simulink model "MPSK_AWGN"  (R2013a)
settings: Solver=ode45  StartTime=0.0  StopTime=10.0  RelTol=1e-3
values from neighbouring files (symbols this model uses):
  EbNodB = EbNoVec(n)    [PSK_AWGN.m]
  M = 8    [PSK_AWGN.m]    (also in SimulatePSK.m = 2.^k; Untitled2.m)
  Tsym = 0.1    [PSK_AWGN.m]
libraries: commsink2 x2, commutil2 x2, commdigbbndpm3 x2, commchan3 x1, commrandsrc2 x1
settings Model: Creator=Administrator  LastModifiedBy=Administrator

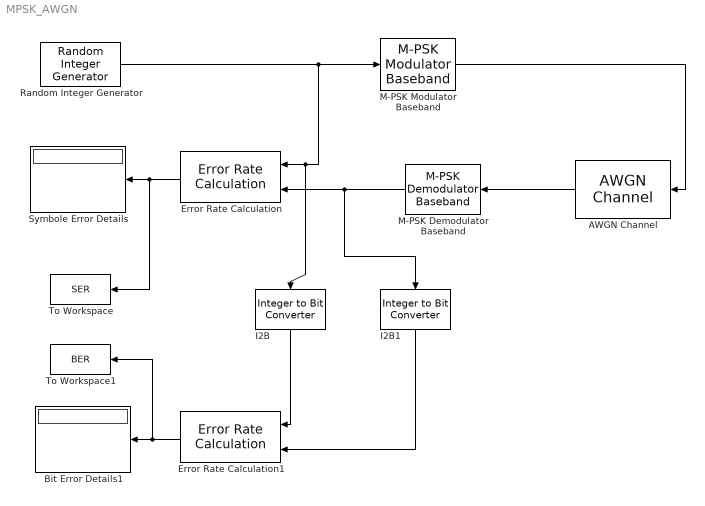
== system MPSK_AWGN ==
  AWGN Channel : commchan3/AWGN Channel  InputProcessing=Columns as channels (frame based)  seed=123456  noiseMode="Signal to noise ratio  (Eb/No)"  EbNodB=EbNodB+10*log10(log2(M))  EsNodB=10  SNRdB=10  bitsPerSym=1  Ps=1  Tsym=Tsym  variance=1
  Bit Error Details1 : Display
      settings: Decimation=3
  Error Rate Calculation : commsink2/Error Rate Calculation  N=1  st_delay=0  cp_mode=Entire frame  subframe=[]  PMode=Port  WsName=ErrorVec  RsMode2=off  stop=off  numErr=100  maxBits=1e6
  Error Rate Calculation1 : commsink2/Error Rate Calculation  N=1  st_delay=0  cp_mode=Entire frame  subframe=[]  PMode=Port  WsName=ErrorVec  RsMode2=off  stop=off  numErr=100  maxBits=1e6
  I2B : commutil2/Integer to Bit Converter  nbits=log2(M)  signedInputValues=Unsigned  bitOrder=MSB first  outDtype=Inherit via internal rule
  I2B1 : commutil2/Integer to Bit Converter  nbits=log2(M)  signedInputValues=Unsigned  bitOrder=MSB first  outDtype=Inherit via internal rule
  M-PSK Demodulator Baseband : commdigbbndpm3/M-PSK Demodulator Baseband  M=8  Ph=pi/8  Dec=Gray  Mapping=[0:7]  OutType=Integer  DecType=Hard decision  VarSource=Dialog  Variance=1  outDtype1=Inherit via internal rule  outDtype2=Inherit via internal rule  derotateFactorWordLen=16
  M-PSK Modulator Baseband : commdigbbndpm3/M-PSK Modulator Baseband  M=8  InType=Integer  Enc=Gray  Mapping=[0:7]  Ph=pi/8  outDtype=double  outWordLen=16  outUDDataType=sfix(16)  outFracLenMode=Best precision  outFracLen=15
  Random Integer Generator : commrandsrc2/Random Integer Generator  mul=M  seed=654321  Ts=Tsym  frameBased=off  sampPerFrame=1  orient=off  outDataType=double
  Symbole Error Details : Display
      settings: Decimation=3
  To Workspace : ToWorkspace  VariableName=SER  SampleTime=-1
  To Workspace1 : ToWorkspace  VariableName=BER  SampleTime=-1
  wires:
  Random Integer Generator/1 -> M-PSK Modulator Baseband/1, Error Rate Calculation/1, I2B/1
  Error Rate Calculation/1 -> To Workspace/1, Symbole Error Details/1
  M-PSK Demodulator Baseband/1 -> I2B1/1, Error Rate Calculation/2
  AWGN Channel/1 -> M-PSK Demodulator Baseband/1
  M-PSK Modulator Baseband/1 -> AWGN Channel/1
  I2B/1 -> Error Rate Calculation1/1
  I2B1/1 -> Error Rate Calculation1/2
  Error Rate Calculation1/1 -> To Workspace1/1, Bit Error Details1/1
